simulink model "dc_motor_model_basic_blocks_feedforward"  (Simulink 7.8)
settings: Solver=ode45  StartTime=0.0  StopTime=10.0  RelTol=1e-3
values from neighbouring files (symbols this model uses):
  J = 8.85*10^(-7)    (= 8.85e-07)    [dc_motor_basic_blocks_feedforward.m]    (also in dc_motor_basic_blocks_feedforward_test.m; dc_motor_h_bridge_feedforward.m)
  k_emf = k_tau    (= 0.0452)    [dc_motor_basic_blocks_feedforward.m]    (also in dc_motor_basic_blocks_feedforward_test.m; dc_motor_h_bridge_feedforward.m)
  k_tau = 0.0452    [dc_motor_basic_blocks_feedforward.m]    (also in dc_motor_basic_blocks_feedforward_test.m; dc_motor_h_bridge_feedforward.m)
  L = 0.746*10^(-3)    (= 0.000746)    [dc_motor_basic_blocks_feedforward.m]    (also in dc_motor_basic_blocks_feedforward_test.m; dc_motor_h_bridge_feedforward.m)
  mu = 10^(-6)    (= 1e-06)    [dc_motor_basic_blocks_feedforward.m]    (also in dc_motor_basic_blocks_feedforward_test.m; dc_motor_h_bridge_feedforward.m)
  R = 7.25    [dc_motor_basic_blocks_feedforward.m]    (also in dc_motor_basic_blocks_feedforward_test.m; dc_motor_h_bridge_feedforward.m)
  T_load = 0.1    [dc_motor_basic_blocks_feedforward.m]    (also in dc_motor_basic_blocks_feedforward_test.m; dc_motor_h_bridge_feedforward.m)
  U_d = (R*mu/k_tau + k_emf) * w_d + R/k_tau * T_load + R*J/k_tau*w_d_dot    (= 34.1839823009)    [dc_motor_basic_blocks_feedforward.m]    (also in dc_motor_basic_blocks_feedforward_test.m; dc_motor_h_bridge_feedforward.m)
settings Model: Creator=krzysztof  LastModifiedBy=krzysztof

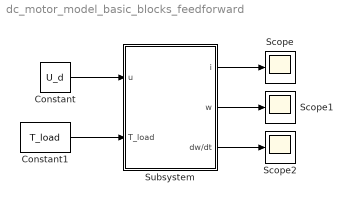
== system dc_motor_model_basic_blocks_feedforward ==
  Constant : Constant  Value=U_d
  Constant1 : Constant  Value=T_load
  Scope : Scope
      settings: SaveName=i_motor
  Scope1 : Scope
      settings: SaveName=w
  Scope2 : Scope
      settings: SaveName=ScopeData2
  Subsystem : Subsystem
  wires:
  Constant/1 -> Subsystem/1(u)
  Constant1/1 -> Subsystem/2(T_load)
  Subsystem/1(i) -> Scope/1
  Subsystem/3(dw/dt) -> Scope2/1
  Subsystem/2(w) -> Scope1/1

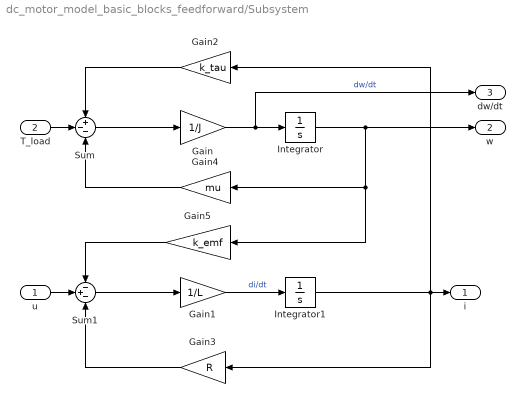
== system dc_motor_model_basic_blocks_feedforward/Subsystem ==
  u : Inport
  T_load : Inport  Port=2
  Gain : Gain  Gain=1/J
  Gain1 : Gain  Gain=1/L
  Gain2 : Gain  Gain=k_tau
  Gain3 : Gain  Gain=R
  Gain4 : Gain  Gain=mu
  Gain5 : Gain  Gain=k_emf
  Integrator : Integrator
  Integrator1 : Integrator
  Sum : Sum  Inputs=+--
  Sum1 : Sum  Inputs=-+-
  i : Outport
  w : Outport  Port=2
  dw/dt : Outport  Port=3
  wires:
  Integrator/1 -> Gain4/1, Gain5/1, w/1
  Integrator1/1 -> Gain2/1, Gain3/1, i/1
  Gain/1 -> Integrator/1, dw/dt/1  "dw/dt"
  Gain1/1 -> Integrator1/1  "di/dt"
  Sum/1 -> Gain/1
  Sum1/1 -> Gain1/1
  Gain2/1 -> Sum/1
  Gain3/1 -> Sum1/3
  Gain4/1 -> Sum/3
  Gain5/1 -> Sum1/1
  T_load/1 -> Sum/2
  u/1 -> Sum1/2
